simulink model "q2_model"  (R2026a)
settings: Solver=VariableStepAuto
values from neighbouring files (symbols this model uses):
  A = [0 1 ... (first row only)    [q2.m]
  B = [gamma ... (first row only)    [q2.m]
  C = [1 0]    [q2.m]
  D = 0    [q2.m]
  K = [k1, k2]    [q2.m]
  kr = k1    (= 1)    [q2.m]
  L = [l1; l2]    [q2.m]
settings Model: Creator=LAB_PC  LastModifiedBy=LAB_PC

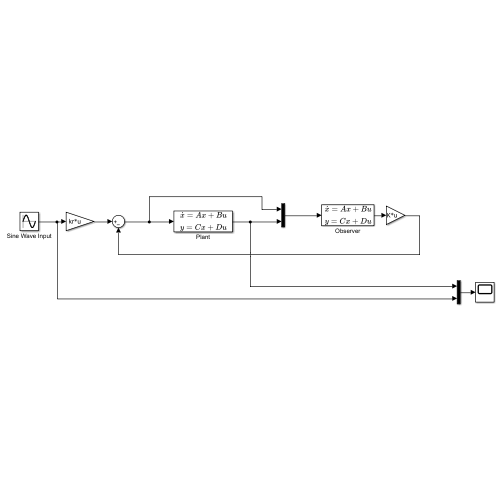
[thumbnail: Simulink's stored preview of the top-level diagram]
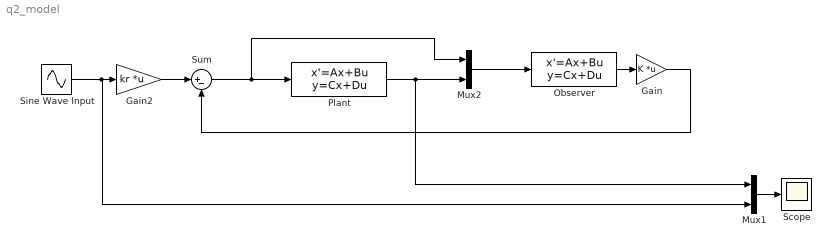
== system q2_model ==
  Gain : Gain  Gain=K  Multiplication=Matrix(K*u)
  Gain2 : Gain  Gain=kr  Multiplication=Matrix(K*u)
  Mux1 : Mux  Inputs=2
  Mux2 : Mux  Inputs=2
  Observer : StateSpace  A=A-L*C  B=[B, L]  C=eye(2)  D=zeros(2,2)  InitialCondition=0
  Plant : StateSpace  A=A  B=B  C=C  D=D  InitialCondition=0
  Scope : Scope
      settings: ActiveDisplayYMinimum=-1.2456318853205086  ActiveDisplayYMaximum=1.2490408795261734
  Sine Wave Input : Sin  SampleTime=0
  Sum : Sum  Inputs=|+-
  wires:
  Sine Wave Input/1 -> Mux1/2, Gain2/1
  Gain2/1 -> Sum/1
  Sum/1 -> Mux2/1, Plant/1
  Plant/1 -> Mux2/2, Mux1/1
  Observer/1 -> Gain/1
  Gain/1 -> Sum/2
  Mux1/1 -> Scope/1
  Mux2/1 -> Observer/1
